simulink library "bcm"  (R2021b)
settings: Solver=VariableStepAuto  StartTime=0.0  StopTime=10.0  RelTol=1e-3
undefined symbols (not defined in the file or in its folder): ENUM_ANTITHEFT_ALARM, ENUM_ANTITHEFT_ARM, ENUM_ANTITHEFT_DISARM, ENUM_ANTITHEFT_WAIT, ENUM_GEARPOSNTOCAN_P, ENUM_PDKEYRAWLULOCK_INUNLOCK, ENUM_PDKEYRAWPS_INPS, ENUM_POWERSTA_READY, ENUM_POWERSTA_STANDBY, FALSE, KBCM_ALMBrightnessDark_enum, KBCM_AmbBlue_enum, KBCM_AmbBreathT_K, KBCM_AmbBreathTOut_K, KBCM_AmbGreen_enum, KBCM_AmbLightUser_enum, KBCM_AmbPreset_enum, KBCM_AmbRed_enum, KBCM_Antitheft_enum_ovrdflg, KBCM_Antitheft_enum_ovrdval, KBCM_APMDoorCtrlSta_flg_ovrdflg, KBCM_APMDoorCtrlSta_flg_ovrdval, KBCM_DelayTSW_flg, KBCM_DiagFLTC_mA, KBCM_DiagFMHT_s, KBCM_DiagFRTC_mA, KBCM_DiagRLTC_mA, KBCM_DiagRRTC_mA, KBCM_DrAPMRetryTimes_cnt, KBCM_DrOpenWdwOT_s, KBCM_DrOpenWdwReady_s, KBCM_ESSOffT_ms, KBCM_ESSOnT_ms, KBCM_IVIRstHoldT_ms, KBCM_IVIRstTriggerT_ms, KBCM_ONDelayT_ms, KBCM_ReDetectT_K, KBCM_RmLampKeep_min, KBCM_RmLpKeyInT_s, KBCM_RmLpKeyMissT_s, KBCM_SlpDebounceTime_s, KBCM_SPTGDetectT_sec, KBCM_SPTGLeave_flg, KBCM_SPTGLeftBound_cm, KBCM_SPTGLeftBoundOut_cm, KBCM_SPTGLowerBound_cm, KBCM_SPTGLowerBoundOut_cm, KBCM_SPTGRightBound_cm, KBCM_SPTGRightBoundOut_cm, KBCM_SPTGTOut_K, KBCM_SPTGUpperBound_cm, KBCM_SPTGUpperBoundOut_cm, KBCM_SPTGWaitDKC_sec, KBCM_USSDis_cm, KBCM_USSFilterT_K, KBCM_WaitAPMPwr_K, KBCM_WdwManualDetT_s, MIN2SEC, TRUE, XX2KXX
libraries: simulink x41, $bdroot x3, hcu_lib x2
(part 2 of 6)

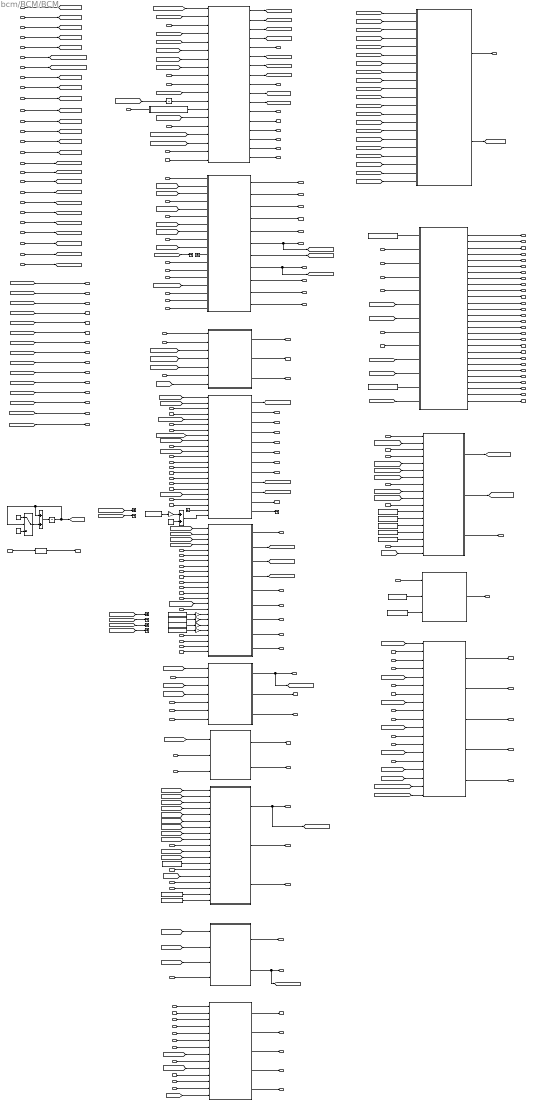
== system bcm/BCM/BCM ==
  task_time_s : Inport
  VINP_VehSpeed_kph : Inport  Port=2
  VINP_AirBagFailCmd_flg : Inport  Port=3
  VINP_ActBrkLampSta_flg : Inport  Port=4
  VINP_SRRODAWarnR_flg : Inport  Port=5
  VINP_SRRODAWarnL_flg : Inport  Port=6
  VINP_SRRBSDWarnR_flg : Inport  Port=7
  VINP_SRRBSDWarnL_flg : Inport  Port=8
  VINP_ESSActive_flg : Inport  Port=9
  VINP_LeftTurnReq_flg : Inport  Port=10
  VINP_RightTurnReq_flg : Inport  Port=11
  VINP_ForceLowBeam_enum : Inport  Port=12
  VINP_HazardWarningReq_flg : Inport  Port=13
  VINP_SetUnlockSingle_flg : Inport  Port=14
  VINP_IVIStatus_flg : Inport  Port=15
  VINP_IVINightModeSta_flg : Inport  Port=16
  VINP_HeadLampSW_enum : Inport  Port=17
  VINP_RFogLampSW_flg : Inport  Port=18
  VINP_FollowMeSW_flg : Inport  Port=19
  VINP_IVIRRDefReq_flg : Inport  Port=20
  VINP_IVIWIMAINSW_flg : Inport  Port=21
  VINP_CANMsgValidIVI2_flg : Inport  Port=22
  VINP_CDLUnlockButt_flg : Inport  Port=23  OutDataTypeStr=boolean
  VINP_CDLLockButt_flg : Inport  Port=24  OutDataTypeStr=boolean
  VINP_RoomLampMode_flg : Inport  Port=25
  VINP_MFRDNBrightReq_pct : Inport  Port=26
  VINP_METERKPHCalcu_kph : Inport  Port=27
  VINP_IVIPWModeReq_enum : Inport  Port=28
  VINP_LINKtoDrive_flg : Inport  Port=29
  VINP_AmbLightColorSet_enum : Inport  Port=30
  VINP_AmbLightUserSet_enum : Inport  Port=31
  VINP_DRAmbLightBrightnessSet_pct : Inport  Port=32
  VINP_IPAmbLightBrightnessSet_pct : Inport  Port=33
  VINP_IVIPTGUSStaSW_flg : Inport  Port=34
  VINP_LDrvControlCommand_pct : Inport  Port=35
  VINP_LPasControlCommand_pct : Inport  Port=36
  VINP_LRLDControlCommand_pct : Inport  Port=37
  VINP_LRRDControlCommand_pct : Inport  Port=38
  VINP_OpenDrOpenWdoSW_flg : Inport  Port=39
  VINP_IVILockSoundSWSta_flg : Inport  Port=40
  VINP_AVMparkingmode_enum : Inport  Port=41
  VINP_CANMsgValidIVI1_flg : Inport  Port=42
  VINP_PCommandToBCM_enum : Inport  Port=43
  VINP_DrLockSta_flg : Inport  Port=44
  VINP_CSWDimSw_flg : Inport  Port=45
  VINP_CSWPassSWSta_flg : Inport  Port=46
  VINP_RLSLampSta_flg : Inport  Port=47
  VINP_CSWTurnSWSta_enum : Inport  Port=48
  VINP_RLTurnLampC_mA : Inport  Port=49
  VINP_RRTurnLampC_mA : Inport  Port=50
  VINP_FLTurnLampC_mA : Inport  Port=51
  VINP_FRTurnLampC_mA : Inport  Port=52
  VINP_MIRRORFOLDSW_flg : Inport  Port=53
  VINP_CSWFWasSWSta_enum : Inport  Port=54
  VINP_CSWFWipSWSta_enum : Inport  Port=55
  VINP_RLSRainSnrWiperCmd_enum : Inport  Port=56
  VINP_FWiperAS_flg : Inport  Port=57
  VINP_CSWRWipIntSwSta_enum : Inport  Port=58
  VINP_RWiperAS_flg : Inport  Port=59
  VINP_CSWRWasSWSta_enum : Inport  Port=60
  VINP_PTGRDILsta_enum : Inport  Port=61
  VINP_RWiperProtection_flg : Inport  Port=62
  VINP_FWiperProtection_flg : Inport  Port=63
  VINP_PDKeyAreaPTG_enum : Inport  Port=64
  VINP_SWCmodeSta_flg : Inport  Port=65
  VINP_CANMsgValidDKC1_flg : Inport  Port=66
  VINP_CANMsgValidGWZoneDR1_flg : Inport  Port=67
  VINP_CANMsgValidGWZoneFR1_flg : Inport  Port=68
  VINP_PTGInnerSW2_enum : Inport  Port=69
  VINP_LDrvValWdwOpened_pct : Inport  Port=70
  VINP_LPasValWdwOpened_pct : Inport  Port=71
  VINP_LRLDValWdwOpened_pct : Inport  Port=72
  VINP_LRRDValWdwOpened_pct : Inport  Port=73
  VINP_PDKeyAreaLockUnlock_enum : Inport  Port=74
  VINP_PDKeyAreaPS_enum : Inport  Port=75
  VINP_ReDoorLock_enum : Inport  Port=76
  VINP_ReOutsideMirror_enum : Inport  Port=77
  VINP_HoodSW_flg : Inport  Port=78
  VINP_TailgateSW_flg : Inport  Port=79
  VINP_DrDoorSW_flg : Inport  Port=80
  VINP_PsDoorSW_flg : Inport  Port=81
  VINP_RLDoorSW_flg : Inport  Port=82
  VINP_RRDoorSW_flg : Inport  Port=83
  VINP_TrunkHanSW_flg : Inport  Port=84
  VINP_HazardSW_flg : Inport  Port=85
  VINP_CentralDoorLockSW_flg : Inport  Port=86
  VINP_BrakeSWGPIO_flg : Inport  Port=87
  VPMM_PwrSta_enum : Inport  Port=88
  VTQD_ShiftGearPosn_enum : Inport  Port=89
  VTQD_CrashDetd_flg : Inport  Port=90
  VTQD_DiagHCrash_flg : Inport  Port=91
  VTQD_ReBrakeLPReq_flg : Inport  Port=92
  VINP_FlashAntitheft_enum : Inport  Port=93
  VINP_FlashCountAlarm_enum : Inport  Port=94
  VINP_FlashMFSWTri_flg : Inport  Port=95
  VINP_FlashMirrorFlodPos : Inport  Port=96
  VINP_FlashFuelDoorPos : Inport  Port=97
  VINP_FlashLockSetting_flg : Inport  Port=98
  VINP_FlashMFRDNBrightReq_pct : Inport  Port=99
  VINP_FlashRoomLampMode_flg : Inport  Port=100
  VINP_FlashWiperFixMode_flg : Inport  Port=101
  VINP_FlashIVIPTGUSStaSW_flg : Inport  Port=102
  VINP_FlashHoodSW_flg : Inport  Port=103
  VINP_FlashTailgateSW_flg : Inport  Port=104
  VINP_FlashCTDLockSW_flg : Inport  Port=105
  VINP_FlashTailgateHDSW_flg : Inport  Port=106
  VINP_FlashAPMDoorControlSta_flg : Inport  Port=107
  VINP_funAuto_flg : Inport  Port=108
  VINP_DiagDRLOFF_flg : Inport  Port=109
  VINP_DiagFMHT_s : Inport  Port=110
  VINP_DiagFLTC_mA : Inport  Port=111
  VINP_DiagFRTC_mA : Inport  Port=112
  VINP_DiagRLTC_mA : Inport  Port=113
  VINP_DiagRRTC_mA : Inport  Port=114
  VINP_FlashfUnlockSingle_flg : Inport  Port=115
  VAPM_PASDRMR_cm : Inport  Port=116
  VAPM_PASDRML_cm : Inport  Port=117
  VINP_APSActive_flg : Inport  Port=118
  VINP_RRDefSta_flg : Inport  Port=119
  VDDM_HVRlyOpCFS_flg : Inport  Port=120
  VDDM_MCUActCFS_flg : Inport  Port=121
  APM_Door : Subsystem
  Add1 : Sum
  AmbientLight : Subsystem
  AntiTheft : Subsystem
  BCM_WAKE_MODULE : Subsystem
  CenterDoorLock : Subsystem
  Constant10 : Constant  Value=KBCM_DelayTSW_flg
  Constant11 : Constant  Value=KBCM_ReDetectT_K
  Constant12 : Constant  Value=KBCM_SPTGDetectT_sec
  Constant13 : Constant  Value=KBCM_SPTGLeave_flg
  Constant14 : Constant  Value=KBCM_RmLampKeep_min
  Constant15 : Constant  Value=KBCM_SPTGWaitDKC_sec
  Constant16 : Constant  Value=0
  Constant17 : Constant
  Constant18 : Constant  Value=KBCM_RmLpKeyInT_s
  Constant19 : Constant  Value=KBCM_RmLpKeyMissT_s
  Constant44 : Constant  Value=KBCM_DiagFMHT_s
  Constant45 : Constant  Value=10
  Constant46 : Constant  Value=KBCM_DiagFLTC_mA
  Constant47 : Constant  Value=KBCM_DiagFRTC_mA
  Constant48 : Constant  Value=KBCM_DiagRLTC_mA
  Constant49 : Constant  Value=KBCM_DiagRRTC_mA
  Constant6 : Constant  Value=KBCM_AmbPreset_enum
  Constant7 : Constant  Value=KBCM_AmbLightUser_enum
  Constant8 : Constant  Value=KBCM_IVIRstHoldT_ms
  Constant9 : Constant  Value=KBCM_IVIRstTriggerT_ms
  Data Type Conversion : DataTypeConversion  OutDataTypeStr=uint8
  Dimmer : Subsystem
  ExteriorLight : Subsystem
  FlasherSignal : Subsystem
  Gain{,2..4} (4 alike) : Gain  Gain=10
  Gain1 : Gain  Gain=5
  Ground : Ground
  Ground1 : Ground
  IVI Reset : Subsystem
  PTG : Subsystem
  PowerMirror : Subsystem
  RearDefogger : Subsystem
  RoomLamp : Subsystem
  Sum : Sum
  Switch : Switch  Criteria=u2 > Threshold
  Tailgate : Subsystem
  Terminator{,1..7} (8 alike) : Terminator
  Unit Delay : UnitDelay  SampleTime=-1  HasFrameUpgradeWarning=on
  Unit Delay1 : UnitDelay  SampleTime=-1  HasFrameUpgradeWarning=on
  Verify : Subsystem
  WasherWiper : Subsystem
  VBCM_AntitheftSta_enum : Outport
  VBCM_TailgateRemote_enum : Outport  Port=2
  VBCM_HornCtrl_flg : Outport  Port=3
  VBCM_AllDoorSW_flg : Outport  Port=4
  VBCM_BCMDoorLockSta_flg : Outport  Port=5
  VBCM_AntitheftSeatFlod_flg : Outport  Port=6
  VBCM_HoodSW_flg : Outport  Port=7
  VBCM_TailgateSW_flg : Outport  Port=8
  VBCM_DrDoorSW_flg : Outport  Port=9
  VBCM_PsDoorSW_flg : Outport  Port=10
  VBCM_RLDoorSW_flg : Outport  Port=11
  VBCM_RRDoorSW_flg : Outport  Port=12
  VBCM_LockSetting_flg : Outport  Port=13
  VBCM_FrChargingDoorCtrl_enum : Outport  Port=14
  VBCM_RrChargingDoorCtrl_enum : Outport  Port=15
  VBCM_CrashSDetd_flg : Outport  Port=16
  VBCM_CTDCtrl_enum : Outport  Port=17
  VBCM_DoorLockIND_flg : Outport  Port=18
  VBCM_CTDLockSW_flg : Outport  Port=19
  VBCM_Dimmer_pct : Outport  Port=20
  VBCM_DimmerEN_flg : Outport  Port=21
  VBCM_PosLamp_flg : Outport  Port=22
  VBCM_LBeam_flg : Outport  Port=23
  VBCM_HBeam_flg : Outport  Port=24
  VBCM_RrFogLamp_flg : Outport  Port=25
  VBCM_BrakeLamp_flg : Outport  Port=26
  VBCM_ReverseLamp_flg : Outport  Port=27
  VBCM_LDRL_flg : Outport  Port=28
  VBCM_RDRL_flg : Outport  Port=29
  VBCM_LBSD_flg : Outport  Port=30
  VBCM_RBSD_flg : Outport  Port=31
  VBCM_HazardSW_flg : Outport  Port=32
  VBCM_LTurnLP_flg : Outport  Port=33
  VBCM_RTurnLP_flg : Outport  Port=34
  VBCM_BCMBuzzerReq_flg : Outport  Port=35
  VBCM_MirrorCtrl_enum : Outport  Port=36
  VBCM_MirrorDefog_flg : Outport  Port=37
  VBCM_RrDefog_flg : Outport  Port=38
  VBCM_RoomLampH_flg : Outport  Port=39
  VBCM_RoomLampL_flg : Outport  Port=40
  VBCM_TrunkRel_flg : Outport  Port=41
  VBCM_TailgateHDSW_flg : Outport  Port=42
  VBCM_FWiperL_flg : Outport  Port=43
  VBCM_FWiperH_flg : Outport  Port=44
  VBCM_RWiper_flg : Outport  Port=45
  VBCM_WasherCtrl_enum : Outport  Port=46
  VBCM_WiperFixMode_flg : Outport  Port=47
  VBCM_SleepReq_flg : Outport  Port=48
  VBCM_User1DrAmbLightBrightness_pct : Outport  Port=49
  VBCM_User1IPAmbLightBrightness_pct : Outport  Port=50
  VBCM_User2DrAmbLightBrightness_enum : Outport  Port=51
  VBCM_User2IPAmbLightBrightness_enum : Outport  Port=52
  VBCM_User3DrAmbLightBrightness_enum : Outport  Port=53
  VBCM_User3IPAmbLightBrightness_enum : Outport  Port=54
  VBCM_User4DrAmbLightBrightness_enum : Outport  Port=55
  VBCM_User4IPAmbLightBrightness_enum : Outport  Port=56
  VBCM_User5DrAmbLightBrightness_enum : Outport  Port=57
  VBCM_User5IPAmbLightBrightness_enum : Outport  Port=58
  VBCM_User6DrAmbLightBrightness_enum : Outport  Port=59
  VBCM_User6IPAmbLightBrightness_enum : Outport  Port=60
  VBCM_User1AmbLightColor_enum : Outport  Port=61
  VBCM_User2AmbLightColor_enum : Outport  Port=62
  VBCM_User3AmbLightColor_enum : Outport  Port=63
  VBCM_User4AmbLightColor_enum : Outport  Port=64
  VBCM_User5AmbLightColor_enum : Outport  Port=65
  VBCM_User6AmbLightColor_enum : Outport  Port=66
  VBCM_AmbLightBreath1_flg : Outport  Port=67
  VBCM_AmbLightBreath2_flg : Outport  Port=68
  VBCM_AmbLightBreath3_flg : Outport  Port=69
  VBCM_AmbLightBrightness1_enum : Outport  Port=70
  VBCM_AmbLightBrightness2_enum : Outport  Port=71
  VBCM_AmbLightBrightness3_enum : Outport  Port=72
  VBCM_AmbLightColor1_enum : Outport  Port=73
  VBCM_AmbLightColor2_enum : Outport  Port=74
  VBCM_AmbLightColor3_enum : Outport  Port=75
  VBCM_LampPwr_flg : Outport  Port=76
  VBCM_SPTGDet_flg : Outport  Port=77
  VBCM_APSOpenPTG_flg : Outport  Port=78
  VBCM_FollowMe_flg : Outport  Port=79
  VBCM_IVIRST_flg : Outport  Port=80
  VBCM_CountAlarm_enum : Outport  Port=81
  VBCM_MFSWTri_flg : Outport  Port=82
  VBCM_MirrorFlodPos_flg : Outport  Port=83
  VBCM_FuelDoorPos_flg : Outport  Port=84
  VBCM_MFRDNBrightReq_pct : Outport  Port=85
  VBCM_RoomLampMode_flg : Outport  Port=86
  VBCM_IVIPTGUSStaSW_flg : Outport  Port=87
  VBCM_PTGInnerSW2_enum : Outport  Port=88
  VBCM_DiagHCrash_flg : Outport  Port=89
  VBCM_DiagFLTS_flg : Outport  Port=90
  VBCM_DiagFRTS_flg : Outport  Port=91
  VBCM_DiagRLTS_flg : Outport  Port=92
  VBCM_DiagRRTS_flg : Outport  Port=93
  VBCM_LDrvCtrlCmd_pct : Outport  Port=94
  VBCM_LPasCtrlCmd_pct : Outport  Port=95
  VBCM_LRLDCtrlCmd_pct : Outport  Port=96
  VBCM_LRRDCtrlCmd_pct : Outport  Port=97
  VBCM_APMDoorControlSta_flg : Outport  Port=98
  VBCM_LockAlarm_enum : Outport  Port=99
  VBCM_ATCtrl_enum : Outport  Port=100
  VBCM_fUnlockSingle_flg : Outport  Port=101
  VBCM_OutMode_enum : Outport  Port=102
  wires:
  VPMM_PwrSta_enum/1 -> [VPMM_PwrSta_enum]
  VINP_TailgateSW_flg/1 -> [VINP_TailgateSW_flg]
  VINP_VehSpeed_kph/1 -> [VINP_VehSpeed_kph]
  AntiTheft/4(VBCM_AntitheftSta_enum) -> [VBCM_AntitheftSta_enum]
  AntiTheft/5(VBCM_TailgateRemote_enum) -> VBCM_TailgateRemote_enum/1
  AntiTheft/6(VBCM_HornCtrl_flg) -> [VBCM_HornCtrl_flg]
  AntiTheft/7(VBCM_AllDoorSW_flg) -> [VBCM_AllDoorSW_flg]
  AntiTheft/9(VBCM_AntitehftSeatFlod_flg) -> VBCM_AntitheftSeatFlod_flg/1
  AntiTheft/8(VBCM_BCMDoorLockSta_flg) -> [VBCM_BCMDoorLockSta_flg]
  AntiTheft/1(VBCM_ATCtrl_enum) -> [VBCM_ATCtrl_enum]
  AntiTheft/2(VBCM_ATActCtrl_enum) -> [VBCM_ATActCtrl_enum]
  AntiTheft/3(VBCM_ATAlarm_flg) -> [VBCM_ATAlarm_flg]
  CenterDoorLock/1(VBCM_LockSetting_flg) -> VBCM_LockSetting_flg/1
  CenterDoorLock/4(VBCM_CrashDetd_flg) -> VBCM_CrashSDetd_flg/1
  VINP_MFRDNBrightReq_pct/1 -> Dimmer/1(VINP_MFRDNBrightReq_pct)
  VINP_IVIStatus_flg/1 -> Dimmer/2(VINP_IVIStatus_flg)
  Dimmer/1(VBCM_Dimmer_pct) -> VBCM_Dimmer_pct/1
  Dimmer/2(VBCM_DimmerEN_flg) -> VBCM_DimmerEN_flg/1
  [VBCM_PosLamp_flg] -> Dimmer/4(VBCM_PosLamp_flag)
  [VPMM_PwrSta_enum] -> PowerMirror/1(VPMM_PwrSta_enum)
  VINP_MIRRORFOLDSW_flg/1 -> PowerMirror/2(VINP_MIRRORFOLDSW_flg)
  [VINP_VehSpeed_kph] -> PowerMirror/3(VINP_VehSpeed_kph)
  [VBCM_ATActCtrl_enum] -> PowerMirror/4(VBCM_ATActCtrl_enum)
  PowerMirror/1(VBCM_MirrorCtrl_enum) -> [VBCM_MirrorCtrl_enum], VBCM_MirrorCtrl_enum/1
  [VPMM_PwrSta_enum] -> RearDefogger/1(VPMM_PwrSta_enum)
  VINP_RRDefSta_flg/1 -> RearDefogger/2(VINP_RRDefSta_flg)
  VINP_IVIRRDefReq_flg/1 -> RearDefogger/3(VINP_IVIRRDefReq_flg)
  RearDefogger/1(VBCM_MirrorDefog_flg) -> VBCM_MirrorDefog_flg/1
  RearDefogger/2(VBCM_RrDefog_flg) -> VBCM_RrDefog_flg/1
  [VPMM_PwrSta_enum] -> RoomLamp/2(VPMM_PwrSta_enum)
  [VBCM_BCMDoorLockSta_flg] -> RoomLamp/3(VBCM_BCMDoorLockSta_flg)
  [VBCM_AllDoorSW_flg] -> RoomLamp/4(VBCM_AllDoorSW_flg)
  [VBCM_AntitheftSta_enum] -> RoomLamp/5(VBCM_AntitheftSta_enum)
  [VPMM_PwrSta_enum] -> Tailgate/1(VPMM_PwrSta_enum)
  [VINP_VehSpeed_kph] -> Tailgate/2(VINP_VehSpeed_kph)
  [VBCM_BCMDoorLockSta_flg] -> Tailgate/3(VBCM_BCMDoorLockSta_flg)
  VINP_TrunkHanSW_flg/1 -> Tailgate/4(VINP_TrunkHandleSwSG08_flg)
  Tailgate/1(VBCM_TrunkRel_flg) -> VBCM_TrunkRel_flg/1
  [VBCM_fVIGHandle_flg] -> Unit Delay/1
  VINP_RoomLampMode_flg/1 -> RoomLamp/10(VINP_RoomLampMode_flg)
  AntiTheft/10(VBCM_HoodSW_flg) -> [VBCM_HoodSW_flg]
  AntiTheft/11(VBCM_TailgateSW_flg) -> [VBCM_TailgateSW_flg]
  AntiTheft/12(VBCM_DrDoorSW_flg) -> VBCM_DrDoorSW_flg/1
  AntiTheft/13(VBCM_PsDoorSW_flg) -> VBCM_PsDoorSW_flg/1
  AntiTheft/14(VBCM_RLDoorSW_flg) -> VBCM_RLDoorSW_flg/1
  AntiTheft/15(VBCM_RRDoorSW_flg) -> VBCM_RRDoorSW_flg/1
  CenterDoorLock/8(VBCM_CTDLockSW_flg) -> [VBCM_CTDLockSW_flg], VBCM_CTDLockSW_flg/1
  Tailgate/2(VBCM_TailgateHDSW_flg) -> [VBCM_TailgateHDSW_flg], VBCM_TailgateHDSW_flg/1
  VINP_CANMsgValidIVI2_flg/1 -> [VINP_CANMsgValidIVI2_flg]
  [VINP_CANMsgValidIVI2_flg] -> RoomLamp/11(VINP_CANMsgValidIVI2_flg)
  [VINP_TailgateSW_flg] -> RoomLamp/12(VINP_TailgateSW_flg)
  CenterDoorLock/10(VBCM_DiagHCrash_flg) -> VBCM_DiagHCrash_flg/1
  [VBCM_ATCtrl_enum] -> FlasherSignal/2(VBCM_ATCtrl_enum)
  [VBCM_ATAlarm_flg] -> FlasherSignal/3(VBCM_ATAlarm_flg)
  [VPMM_PwrSta_enum] -> FlasherSignal/4(VPMM_PwrSta_enum)
  VINP_HazardSW_flg/1 -> FlasherSignal/5(VINP_HazardSW_flg)
  VINP_CSWTurnSWSta_enum/1 -> FlasherSignal/6(VINP_CSWTurnSWSta_enum)
  VINP_RLTurnLampC_mA/1 -> FlasherSignal/7(VINP_RLTurnLampC_mA)
  VINP_RRTurnLampC_mA/1 -> FlasherSignal/8(VINP_RRTurnLampC_mA)
  VINP_FLTurnLampC_mA/1 -> FlasherSignal/9(VINP_FLTurnLampC_mA)
  VINP_FRTurnLampC_mA/1 -> FlasherSignal/10(VINP_FRTurnLampC_mA)
  VINP_PTGRDILsta_enum/1 -> FlasherSignal/11(VINP_PTGRDILsta_enum)
  VINP_ESSActive_flg/1 -> FlasherSignal/12(VINP_ESSActive_flg)
  VINP_LeftTurnReq_flg/1 -> FlasherSignal/13(VINP_LeftTurnReq_flg)
  VINP_RightTurnReq_flg/1 -> FlasherSignal/14(VINP_RightTurnReq_flg)
  VINP_HazardWarningReq_flg/1 -> FlasherSignal/16(HazardWarningReq)
  FlasherSignal/1(VBCM_HazardSW_flg) -> VBCM_HazardSW_flg/1
  FlasherSignal/2(VBCM_LTurnLP_flg) -> [VBCM_LTurnLP_flg]
  task_time_s/1 -> [task_time_s]
  [VBCM_HoodSW_flg] -> BCM_WAKE_MODULE/1(VBCM_HoodSW_flg)
  [VBCM_TailgateSW_flg] -> BCM_WAKE_MODULE/2(VBCM_TailgateSW_flg)
  [VBCM_CTDLockSW_flg] -> BCM_WAKE_MODULE/3(VBCM_CTDLockSW_flg)
  [VBCM_TailgateHDSW_flg] -> BCM_WAKE_MODULE/4(VBCM_TailgateHDSW_flg)
  [VBCM_AntitheftSta_enum] -> BCM_WAKE_MODULE/5(VBCM_AntitheftSta_enum)
  [VBCM_AllDoorSW_flg] -> BCM_WAKE_MODULE/6(VBCM_AllDoorSW_flg)
  [VBCM_HornCtrl_flg] -> BCM_WAKE_MODULE/7(VBCM_HornCtrl_flg)
  [VBCM_DoorLockIND_flg] -> BCM_WAKE_MODULE/8(VBCM_DoorLockIND_flg)
  [VINP_BrakeSWGPIO_flg] -> BCM_WAKE_MODULE/9(VINP_BrakeSWGPIO_flg)
  [VBCM_PosLamp_flg] -> BCM_WAKE_MODULE/10(VBCM_PosLamp_flg)
  [VBCM_LBSD_flg] -> BCM_WAKE_MODULE/11(VBCM_LBSD_flg)
  [VBCM_RBSD_flg] -> BCM_WAKE_MODULE/12(VBCM_RBSD_flg)
  [VBCM_RTurnLP_flg] -> BCM_WAKE_MODULE/14(VBCM_RTurnLP_flg)
  [VBCM_LTurnLP_flg] -> BCM_WAKE_MODULE/13(VBCM_LTurnLP_flg)
  [VBCM_MirrorCtrl_enum] -> BCM_WAKE_MODULE/15(VBCM_MirrorCtrl_enum)
  [VBCM_RoomLampH_flg] -> BCM_WAKE_MODULE/16(VBCM_RoomLampH_flg)
  [task_time_s] -> BCM_WAKE_MODULE/17(task_time_s)
  BCM_WAKE_MODULE/1(VBCM_SleepReq_flg) -> VBCM_SleepReq_flg/1
  [VPMM_PwrSta_enum] -> ExteriorLight/2(VPMM_PwrSta_enum)
  VINP_ForceLowBeam_enum/1 -> ExteriorLight/18(VINP_ForceLowBeam_enum)
  VTQD_ReBrakeLPReq_flg/1 -> ExteriorLight/20(VTQD_ReBrakeLPReq_flg)
  VINP_METERKPHCalcu_kph/1 -> ExteriorLight/21(VINP_METERKPHCalcu_kph)
  VINP_SRRBSDWarnL_flg/1 -> ExteriorLight/17(VINP_SRRBSDWarnL_flg)
  VINP_SRRBSDWarnR_flg/1 -> ExteriorLight/16(VINP_SRRBSDWarnR_flg)
  VINP_SRRODAWarnL_flg/1 -> ExteriorLight/15(VINP_SRRODAWarnL_flg)
  VINP_SRRODAWarnR_flg/1 -> ExteriorLight/14(VINP_SRRODAWarnR_flg)
  VINP_ActBrkLampSta_flg/1 -> ExteriorLight/13(VINP_ActBrkLampSta_flg)
  VINP_RLSLampSta_flg/1 -> ExteriorLight/12(VINP_RLSLampSta_flg)
  VINP_FollowMeSW_flg/1 -> ExteriorLight/10(VINP_FollowMeSW_flg)
  VINP_CSWPassSWSta_flg/1 -> ExteriorLight/7(VINP_CSWPassSWSta_flg)
  VINP_CSWDimSw_flg/1 -> ExteriorLight/6(VINP_CSWDimSw_flg)
  VINP_RFogLampSW_flg/1 -> ExteriorLight/4(VINP_RFogLampSW_flg)
  VINP_HeadLampSW_enum/1 -> ExteriorLight/3(VINP_HeadLampSW_enum)
  [VINP_CANMsgValidIVI2_flg] -> ExteriorLight/19(VINP_CANMsgValidIVI2_flg)
  [VBCM_ATCtrl_enum] -> ExteriorLight/11(VBCM_ATCtrl_enum)
  [VBCM_OutMode_enum] -> ExteriorLight/9(VBCM_OutMode_enum)
  VINP_BrakeSWGPIO_flg/1 -> [VINP_BrakeSWGPIO_flg]
  [VINP_BrakeSWGPIO_flg] -> ExteriorLight/5(VINP_BrakeSWGPIO_flg)
  ExteriorLight/2(VBCM_LBeam_flg) -> VBCM_LBeam_flg/1
  ExteriorLight/3(VBCM_HBeam_flg) -> VBCM_HBeam_flg/1
  ExteriorLight/1(VBCM_PosLamp_flg) -> [VBCM_PosLamp_flg]
  ExteriorLight/4(VBCM_RrFogLamp_flg) -> VBCM_RrFogLamp_flg/1
  ExteriorLight/5(VBCM_BrakeLamp_flg) -> VBCM_BrakeLamp_flg/1
  ExteriorLight/6(VBCM_ReverseLamp_flg) -> VBCM_ReverseLamp_flg/1
  ExteriorLight/7(VBCM_LDRL_flg) -> VBCM_LDRL_flg/1
  ExteriorLight/8(VBCM_RDRL_flg) -> VBCM_RDRL_flg/1
  ExteriorLight/10(VBCM_RBSD_flg) -> [VBCM_RBSD_flg]
  ExteriorLight/9(VBCM_LBSD_flg) -> [VBCM_LBSD_flg]
  ExteriorLight/12(VBCM_showup_flg) -> Terminator5/1
  VINP_DrDoorSW_flg/1 -> [VINP_DrDoorSW_flg]
  VINP_IVINightModeSta_flg/1 -> [VINP_IVINightModeSta_flg]
  [VINP_IVINightModeSta_flg] -> Dimmer/3(VINP_IVINightModeSta_flg)
  [VBCM_AntitheftSta_enum] -> VBCM_AntitheftSta_enum/1
  [VBCM_HornCtrl_flg] -> VBCM_HornCtrl_flg/1
  [VBCM_AllDoorSW_flg] -> VBCM_AllDoorSW_flg/1
  [VBCM_BCMDoorLockSta_flg] -> VBCM_BCMDoorLockSta_flg/1
  [VBCM_HoodSW_flg] -> VBCM_HoodSW_flg/1
  [VBCM_TailgateSW_flg] -> VBCM_TailgateSW_flg/1
  [VINP_CANMsgValidIVI2_flg] -> Dimmer/5(VINP_CANMsgValidIVI2_flg)
  VINP_ReOutsideMirror_enum/1 -> PowerMirror/5(VINP_ReOutsideMirror_enum)
  AmbientLight/1(VBCM_User1DrAmbLightBrightness_enum) -> VBCM_User1DrAmbLightBrightness_pct/1
  AmbientLight/2(VBCM_User1IPAmbLightBrightness_enum) -> VBCM_User1IPAmbLightBrightness_pct/1
  AmbientLight/3(VBCM_User2DrAmbLightBrightness_enum) -> VBCM_User2DrAmbLightBrightness_enum/1
  AmbientLight/4(VBCM_User2IPAmbLightBrightness_enum) -> VBCM_User2IPAmbLightBrightness_enum/1
  AmbientLight/5(VBCM_User3DrAmbLightBrightness_enum) -> VBCM_User3DrAmbLightBrightness_enum/1
  AmbientLight/6(VBCM_User3IPAmbLightBrightness_enum) -> VBCM_User3IPAmbLightBrightness_enum/1
  AmbientLight/7(VBCM_User4DrAmbLightBrightness_enum) -> VBCM_User4DrAmbLightBrightness_enum/1
  AmbientLight/8(VBCM_User4IPAmbLightBrightness_enum) -> VBCM_User4IPAmbLightBrightness_enum/1
  AmbientLight/9(VBCM_User5DrAmbLightBrightness_enum) -> VBCM_User5DrAmbLightBrightness_enum/1
  AmbientLight/10(VBCM_User5IPAmbLightBrightness_enum) -> VBCM_User5IPAmbLightBrightness_enum/1
  AmbientLight/11(VBCM_User6DrAmbLightBrightness_enum) -> VBCM_User6DrAmbLightBrightness_enum/1
  AmbientLight/12(VBCM_User6IPAmbLightBrightness_enum) -> VBCM_User6IPAmbLightBrightness_enum/1
  AmbientLight/13(VBCM_User1AmbLightColor_enum) -> VBCM_User1AmbLightColor_enum/1
  AmbientLight/14(VBCM_User2AmbLightColor_enum) -> VBCM_User2AmbLightColor_enum/1
  AmbientLight/15(VBCM_User3AmbLightColor_enum) -> VBCM_User3AmbLightColor_enum/1
  AmbientLight/16(VBCM_User4AmbLightColor_enum) -> VBCM_User4AmbLightColor_enum/1
  AmbientLight/17(VBCM_User5AmbLightColor_enum) -> VBCM_User5AmbLightColor_enum/1
  AmbientLight/18(VBCM_User6AmbLightColor_enum) -> VBCM_User6AmbLightColor_enum/1
  BCM_WAKE_MODULE/2(VBCM_WakeUp_flg) -> [VBCM_WakeUp_flg]
  [VPMM_PwrSta_enum] -> AmbientLight/10(VPMM_PwrSta_enum)
  [VBCM_PosLamp_flg] -> AmbientLight/11(VBCM_PosLamp_flg)
  [VINP_DrDoorSW_flg] -> AmbientLight/7(VINP_DrDoorSW_flg)
  Constant6/1 -> AmbientLight/12(KBCM_AmbPreset_enum)
  VINP_AmbLightUserSet_enum/1 -> AmbientLight/2(VINP_AmbLightUserSet_enum)
  VINP_AmbLightColorSet_enum/1 -> AmbientLight/3(VINP_AmbLightColorSet_enum)
  VINP_LINKtoDrive_flg/1 -> AmbientLight/4(VINP_LINKtoDrive_flg)
  VINP_IPAmbLightBrightnessSet_pct/1 -> AmbientLight/8(VINP_IPAmbLightBrightnessSet_enum)
  VINP_DRAmbLightBrightnessSet_pct/1 -> AmbientLight/9(VINP_DrAmbLightBrightnessSet_enum)
  Constant7/1 -> AmbientLight/1(VINP_AmbLightUser_enum)
  [VBCM_WakeUp_flg] -> AmbientLight/13(VBCM_WakeUp_flg)
  AmbientLight/19(VBCM_AmbLightBreath1_flg) -> VBCM_AmbLightBreath1_flg/1
  AmbientLight/20(VBCM_AmbLightBreath2_flg) -> VBCM_AmbLightBreath2_flg/1
  AmbientLight/21(VBCM_AmbLightBreath3_flg) -> VBCM_AmbLightBreath3_flg/1
  AmbientLight/22(VBCM_AmbLightBrightness1_enum) -> VBCM_AmbLightBrightness1_enum/1
  AmbientLight/23(VBCM_AmbLightBrightness2_enum) -> VBCM_AmbLightBrightness2_enum/1
  AmbientLight/24(VBCM_AmbLightBrightness3_enum) -> VBCM_AmbLightBrightness3_enum/1
  AmbientLight/25(VBCM_AmbLightColor1_enum) -> VBCM_AmbLightColor1_enum/1
  AmbientLight/26(VBCM_AmbLightColor2_enum) -> VBCM_AmbLightColor2_enum/1
  AmbientLight/27(VBCM_AmbLightColor3_enum) -> VBCM_AmbLightColor3_enum/1
  AmbientLight/28(VBCM_LampPwr_flg) -> VBCM_LampPwr_flg/1
  VINP_IVIPWModeReq_enum/1 -> AmbientLight/5(VINP_IVIPWModeReq_enum)
  [VINP_IVINightModeSta_flg] -> AmbientLight/6(VINP_IVINightModeSta_flg)
  VINP_FlashAntitheft_enum/1 -> Verify/1(VINP_FlashAntitheft_enum)
  [VPMM_PwrSta_enum] -> WasherWiper/8(VPMM_PwrSta_enum)
  [VINP_CANMsgValidIVI2_flg] -> WasherWiper/10(VINP_CANMsgValidIVI2_flg)
  VINP_FWiperProtection_flg/1 -> WasherWiper/12(VINP_FWiperProtection_flg)
  VINP_CSWFWasSWSta_enum/1 -> WasherWiper/1(VINP_CSWFWasSWSta_enum)
  VINP_CSWFWipSWSta_enum/1 -> WasherWiper/2(VINP_CSWFWipSWSta_enum)
  VINP_RLSRainSnrWiperCmd_enum/1 -> WasherWiper/3(VINP_RLSRainSnrWiperCmd_enum)
  VINP_FWiperAS_flg/1 -> WasherWiper/4(VINP_FWiperAS_flg)
  VINP_CSWRWipIntSwSta_enum/1 -> WasherWiper/5(VINP_CSWRWipIntSwSta_enum)
  VINP_RWiperAS_flg/1 -> WasherWiper/6(VINP_RWiperAS_flg)
  VINP_CSWRWasSWSta_enum/1 -> WasherWiper/7(VINP_CSWRWasSWSta_enum)
  VINP_IVIWIMAINSW_flg/1 -> WasherWiper/9(VINP_IVIWIMAINSW_flg)
  VINP_RWiperProtection_flg/1 -> WasherWiper/11(VINP_RWiperProtection_flg)
  WasherWiper/1(VBCM_FrWiperL_flg) -> VBCM_FWiperL_flg/1
  WasherWiper/2(VBCM_FrWiperH_flg) -> VBCM_FWiperH_flg/1
  WasherWiper/3(VBCM_RrWiper_flg) -> VBCM_RWiper_flg/1
  WasherWiper/4(VBCM_WasherCtrl_enum) -> VBCM_WasherCtrl_enum/1
  WasherWiper/5(VBCM_WiperFixMode_flg) -> VBCM_WiperFixMode_flg/1
  PTG/2(VBCM_APSOpenPTG_flg) -> [VBCM_APSOpenPTG_flg]  "VBCM_APSOpenPTG_flg"
  [VTQD_ShiftGearPosn_enum] -> PTG/7(VTQD_ShiftGearPosn_enum)
  [VPMM_PwrSta_enum] -> PTG/6(VPMM_PwrSta_eunm)
  [VINP_VehSpeed_kph] -> PTG/10(VINP_VehSpeed_kph)
  PTG/1(VBCM_SPTGDet_flg) -> [VBCM_SPTGDet_flg]  "VBCM_SPTGDet_flg"
  VAPM_PASDRMR_cm/1 -> PTG/3(VAPM_PASDRMR_cm)
  VAPM_PASDRML_cm/1 -> PTG/4(VAPM_PASDRML_cm)
  [VINP_CANMsgValidIVI2_flg] -> PTG/9(VINP_CANMsgValidIVI2_flg)
  [VINP_PCommandToBCM_enum] -> PTG/5(VINP_PCommandToBCM_enum)
  [VINP_TailgateSW_flg] -> PTG/2(VINP_TailgateSW_flg)
  VINP_PDKeyAreaPTG_enum/1 -> PTG/1(VINP_PDKeyAreaPTG_enum)
  VINP_IVIPTGUSStaSW_flg/1 -> PTG/8(VINP_IVIPTGUSStaSW_flg)
  [VBCM_SPTGDet_flg] -> FlasherSignal/15(VINP_SPTGDet_flg)
  VTQD_ShiftGearPosn_enum/1 -> [VTQD_ShiftGearPosn_enum]
  [VTQD_ShiftGearPosn_enum] -> ExteriorLight/8(VTQD_ShiftGearPosn_enum)
  VINP_PCommandToBCM_enum/1 -> [VINP_PCommandToBCM_enum]
  Constant8/1 -> IVI Reset/2(KBCM_IVIRstHoldT_ms)
  Constant9/1 -> IVI Reset/3(KBCM_IVIRstTriggerT_ms)
  VINP_SWCmodeSta_flg/1 -> IVI Reset/1(VINP_SWCmodeSta_flg)
  IVI Reset/1(VBCM_IVIRST_flg) -> VBCM_IVIRST_flg/1
  [VBCM_APSOpenPTG_flg] -> VBCM_APSOpenPTG_flg/1
  [VBCM_SPTGDet_flg] -> VBCM_SPTGDet_flg/1
  [VBCM_PosLamp_flg] -> VBCM_PosLamp_flg/1
  ExteriorLight/11(VBCM_FollowMe_flg) -> VBCM_FollowMe_flg/1
  [VBCM_LBSD_flg] -> VBCM_LBSD_flg/1
  [VBCM_RBSD_flg] -> VBCM_RBSD_flg/1
  [VBCM_LTurnLP_flg] -> VBCM_LTurnLP_flg/1
  [VBCM_RTurnLP_flg] -> VBCM_RTurnLP_flg/1
  VDDM_MCUActCFS_flg/1 -> FlasherSignal/22(VDDM_MCUActCFS_flg)
  VDDM_HVRlyOpCFS_flg/1 -> FlasherSignal/21(VDDM_HVRlyOpCFS_flg)
  Constant14/1 -> RoomLamp/13(KBCM_RmLampKeep_min)
  VINP_FlashMFSWTri_flg/1 -> PowerMirror/6(EEP_MFSWTri_flg)
  VINP_FlashMirrorFlodPos/1 -> PowerMirror/7(EEP_MirrorFlodPos)
  PowerMirror/2(MFSWTri) -> VBCM_MFSWTri_flg/1
  PowerMirror/3(MirrorFlodPos) -> VBCM_MirrorFlodPos_flg/1
  CenterDoorLock/9(VBCM_FuelDoorPos_flg) -> VBCM_FuelDoorPos_flg/1
  AntiTheft/16(VBCM_CountAlarm_enum) -> VBCM_CountAlarm_enum/1
  Constant10/1 -> PTG/12(KBCM_DelayTSW_flg)
  Constant11/1 -> PTG/13(KBCM_ReDetectT_K)
  Constant12/1 -> PTG/14(KBCM_SPTGDetectT_sec)
  Constant13/1 -> PTG/15(KBCM_SPTGLeave_flg)
  Constant15/1 -> PTG/16(KBCM_SPTGWaitDKC_sec)
  VINP_CANMsgValidDKC1_flg/1 -> PTG/11(VINP_CANMsgValidDKC1_flg)
  VINP_FlashMFRDNBrightReq_pct/1 -> Dimmer/6(EEP_MFRDNBrightReq)
  VINP_FlashRoomLampMode_flg/1 -> RoomLamp/14(EEP_RoomLampMode)
  VINP_FlashWiperFixMode_flg/1 -> WasherWiper/13(VINP_FlashWiperFixMode)
  Dimmer/3(VBCM_MFRDNBrightReq_pct) -> VBCM_MFRDNBrightReq_pct/1
  Sum/1 -> Unit Delay1/1
  Switch/1 -> Sum/2
  Constant17/1 -> Switch/3
  Constant16/1 -> Switch/1
  Unit Delay1/1 -> [BCMInitial], Switch/2, Sum/1
  [BCMInitial] -> WasherWiper/14(BCMInitial)
  [BCMInitial] -> RoomLamp/15(BCMInitial)
  [BCMInitial] -> Dimmer/7(BCMInitial)
  [BCMInitial] -> PTG/18(BCMInitial)
  VINP_FlashIVIPTGUSStaSW_flg/1 -> PTG/17(EEP_IVIPTGUSStaSW)
  PTG/3(VBCM_IVIPTGUSStaSW_flg) -> VBCM_IVIPTGUSStaSW_flg/1
  Data Type Conversion/1 -> VBCM_PTGInnerSW2_enum/1  "VBCM_PTGInnerSW2_enum"
  VINP_PTGInnerSW2_enum/1 -> Data Type Conversion/1
  VINP_FlashHoodSW_flg/1 -> [VINP_FlashHoodSW_flg]
  VINP_FlashTailgateSW_flg/1 -> [VINP_FlashTailgateSW_flg]
  VINP_FlashCTDLockSW_flg/1 -> [VINP_FlashCTDLockSW_flg]
  VINP_FlashTailgateHDSW_flg/1 -> [VINP_FlashTailgateHDSW_flg]
  [VINP_FlashHoodSW_flg] -> BCM_WAKE_MODULE/18(VINP_FlashHoodSW_flg)
  [VINP_FlashTailgateSW_flg] -> BCM_WAKE_MODULE/19(VINP_FlashTailgateSW_flg)
  [VINP_FlashCTDLockSW_flg] -> BCM_WAKE_MODULE/20(VINP_FlashCTDLockSW_flg)
  [VINP_FlashTailgateHDSW_flg] -> BCM_WAKE_MODULE/21(VINP_FlashTailgateHDSW_flg)
  [VINP_CANMsgValidGWZoneDR1_flg] -> APM_Door/18(VINP_CANMsgValidGWZoneDR1_flg)
  [VINP_CANMsgValidGWZoneFR1_flg] -> APM_Door/19(VINP_CANMsgValidGWZoneFR1_flg)
  APM_Door/4(VBCM_LRRDCtrlCmd_pct) -> VBCM_LRRDCtrlCmd_pct/1
  APM_Door/2(VBCM_LPasCtrlCmd_pct) -> VBCM_LPasCtrlCmd_pct/1
  APM_Door/3(VBCM_LRLDCtrlCmd_pct) -> VBCM_LRLDCtrlCmd_pct/1
  [VINP_RLDoorSW_flg] -> APM_Door/11(VINP_RLDoorSW_flg)
  [VINP_DrDoorSW_flg] -> APM_Door/5(VINP_DrDoorSW_flg)
  APM_Door/5(VBCM_APMDoorControlSta_flg) -> VBCM_APMDoorControlSta_flg/1
  VINP_LRRDValWdwOpened_pct/1 -> APM_Door/13(VINP_LRRDValWdwOpened_pct)
  [VINP_CANMsgValidIVI2_flg] -> APM_Door/17(VINP_CANMsgValidIVI2_flg)
  [task_time_s] -> APM_Door/1(task_time_s)
  VINP_FlashAPMDoorControlSta_flg/1 -> APM_Door/15(VINP_FlashAPMDoorControlSta_flg)
  VINP_LPasControlCommand_pct/1 -> APM_Door/6(VINP_LPasControlCommand_pct)
  VINP_OpenDrOpenWdoSW_flg/1 -> APM_Door/2(VINP_OpenDrOpenWdoSW_flg)
  VINP_LDrvValWdwOpened_pct/1 -> APM_Door/4(VINP_LDrvValWdwOpened_pct)
  VINP_LPasValWdwOpened_pct/1 -> APM_Door/7(VINP_LPasValWdwOpened_pct)
  VINP_LRLDControlCommand_pct/1 -> APM_Door/9(VINP_LRLDControlCommand_pct)
  VINP_LRRDControlCommand_pct/1 -> APM_Door/12(VINP_LRRDControlCommand_pct)
  APM_Door/1(VBCM_LDrvCtrlCmd_pct) -> VBCM_LDrvCtrlCmd_pct/1
  [VINP_RRDoorSW_flg] -> APM_Door/14(VINP_RRDoorSW_flg)
  [VINP_PsDoorSW_flg] -> APM_Door/8(VINP_PsDoorSW_flg)
  VINP_LRLDValWdwOpened_pct/1 -> APM_Door/10(VINP_LRLDValWdwOpened_pct)
  [BCMInitial] -> APM_Door/16(BCMInitial)
  VINP_LDrvControlCommand_pct/1 -> APM_Door/3(VINP_LDrvControlCommand_pct)
  VINP_PsDoorSW_flg/1 -> [VINP_PsDoorSW_flg]
  VINP_RLDoorSW_flg/1 -> [VINP_RLDoorSW_flg]
  VINP_RRDoorSW_flg/1 -> [VINP_RRDoorSW_flg]
  VINP_CANMsgValidGWZoneDR1_flg/1 -> [VINP_CANMsgValidGWZoneDR1_flg]
  VINP_CANMsgValidGWZoneFR1_flg/1 -> [VINP_CANMsgValidGWZoneFR1_flg]
  RoomLamp/1(VBCM_RoomLampH_flg) -> [VBCM_RoomLampH_flg], VBCM_RoomLampH_flg/1
  RoomLamp/2(VBCM_RoomLampL_flg) -> VBCM_RoomLampL_flg/1
  RoomLamp/3(VBCM_RoomLampMode_flg) -> VBCM_RoomLampMode_flg/1
  [task_time_s] -> RoomLamp/1(task_time_s)
  [VINP_DrDoorSW_flg] -> RoomLamp/6(VINP_DrDoorSW_flg)
  [VINP_PsDoorSW_flg] -> RoomLamp/7(VINP_PsDoorSW_flg)
  [VINP_RLDoorSW_flg] -> RoomLamp/8(VINP_RLDoorSW_flg)
  [VINP_RRDoorSW_flg] -> RoomLamp/9(VINP_RRDoorSW_flg)
  Constant18/1 -> RoomLamp/18(KBCM_RmLpKeyInT_s)  "2400"
  VINP_PDKeyAreaLockUnlock_enum/1 -> RoomLamp/16(VINP_PDKeyAreaLockUnlock_enum)
  Constant19/1 -> RoomLamp/19(KBCM_RmLpKeyMissT_s)  "600"
  VINP_PDKeyAreaPS_enum/1 -> RoomLamp/17(VINP_PDKeyAreaPS_enum)
  VINP_DiagFLTC_mA/1 -> [VINP_DiagFLTC_mA]
  VINP_DiagFRTC_mA/1 -> [VINP_DiagFRTC_mA]
  VINP_DiagRLTC_mA/1 -> [VINP_DiagRLTC_mA]
  VINP_DiagRRTC_mA/1 -> [VINP_DiagRRTC_mA]
  VINP_funAuto_flg/1 -> [VINP_funAuto_flg]
  VINP_DiagDRLOFF_flg/1 -> [VINP_DiagDRLOFF_flg]
  VINP_DiagFMHT_s/1 -> [VINP_DiagFMHT_s]
  [task_time_s] -> ExteriorLight/1(task_time_s)
  FlasherSignal/3(VBCM_RTurnLP_flg) -> [VBCM_RTurnLP_flg]
  FlasherSignal/4(VBCM_OutMode_enum) -> [VBCM_OutMode_enum]
  FlasherSignal/5(VBCM_BCMBuzzerReq_flg) -> VBCM_BCMBuzzerReq_flg/1
  FlasherSignal/6(VBCM_DiagFLTS_flg) -> VBCM_DiagFLTS_flg/1
  FlasherSignal/7(VBCM_DiagFRTS_flg) -> VBCM_DiagFRTS_flg/1
  FlasherSignal/8(VBCM_DiagRLTS_flg) -> VBCM_DiagRLTS_flg/1
  FlasherSignal/9(VBCM_DiagRRTS_flg) -> VBCM_DiagRRTS_flg/1
  VINP_APSActive_flg/1 -> FlasherSignal/23(VINP_APSActive_flg)
  VINP_AVMparkingmode_enum/1 -> FlasherSignal/24(VINP_AVMparkingmode_enum)
  [VBCM_ATCtrl_enum] -> VBCM_ATCtrl_enum/1  "VBCM_ATCtrl_enum"
  Verify/1(VBCM_FlashAntitheft_enum) -> AntiTheft/13(VBCM_FlashAntitheft_enum)  "VBCM_FlashAntitheft_enum"
  [VINP_PCommandToBCM_enum] -> AntiTheft/1(VINP_PCommandToBCM_enum)
  [VPMM_PwrSta_enum] -> AntiTheft/2(VPMM_PwrSta_enum)
  [VINP_TailgateSW_flg] -> AntiTheft/4(VINP_TailgateSW_flg)
  [VINP_DrDoorSW_flg] -> AntiTheft/5(VINP_DrDoorSW_flg)
  [VINP_VehSpeed_kph] -> AntiTheft/11(VINP_VehSpeed_kph)
  [VBCM_APSOpenPTG_flg] -> AntiTheft/14(VINP_APSOpenPTG_flg)
  [VINP_CANMsgValidGWZoneDR1_flg] -> AntiTheft/16(VINP_CANMsgValidGWZoneDR1_flg)
  [VINP_CANMsgValidGWZoneFR1_flg] -> AntiTheft/17(VINP_CANMsgValidGWZoneFR1_flg)
  [VINP_PsDoorSW_flg] -> AntiTheft/6(VINP_PsDoorSW_flg)
  [VINP_RLDoorSW_flg] -> AntiTheft/7(VINP_RLDoorSW_flg)
  [VINP_RRDoorSW_flg] -> AntiTheft/8(VINP_RRDoorSW_flg)
  Unit Delay/1 -> AntiTheft/12(VBCM_fVIGHandle_flg)
  VINP_HoodSW_flg/1 -> AntiTheft/3(VINP_HoodSW_flg)
  VINP_DrLockSta_flg/1 -> AntiTheft/9(VINP_DrLockSta_flg)
  VINP_ReDoorLock_enum/1 -> AntiTheft/10(VINP_ReDoorLock_enum)
  VINP_FlashCountAlarm_enum/1 -> AntiTheft/15(VINP_FlashCountAlarm_enum)
  AntiTheft/17(VBCM_LockAlarm_enum) -> VBCM_LockAlarm_enum/1
  VINP_IVILockSoundSWSta_flg/1 -> AntiTheft/19(VINP_IVILockSoundSWSta_flg)
  VINP_CANMsgValidIVI1_flg/1 -> AntiTheft/18(VINP_CANMsgValidIVI1_flg)
  [VINP_CANMsgValidIVI2_flg] -> CenterDoorLock/15(VINP_CANMsgValidIVI2_flg)
  [VBCM_AntitheftSta_enum] -> CenterDoorLock/2(VBCM_AntitheftSta_enum)
  [VBCM_AllDoorSW_flg] -> CenterDoorLock/3(VBCM_AllDoorSW_flg)
  [VPMM_PwrSta_enum] -> CenterDoorLock/5(VPMM_PwrSta_enum)
  [VBCM_BCMDoorLockSta_flg] -> CenterDoorLock/7(VBCM_BCMDoorLockSta_flg)
  [VBCM_ATActCtrl_enum] -> CenterDoorLock/8(VBCM_ATActCtrl_enum)
  [VINP_VehSpeed_kph] -> CenterDoorLock/10(VINP_VehSpeed_kph)
  VINP_SetUnlockSingle_flg/1 -> CenterDoorLock/1(VINP_SetUnlockSingle_flg)
  VTQD_DiagHCrash_flg/1 -> CenterDoorLock/4(VTQD_DiagHCrash_flg)
  VINP_CentralDoorLockSW_flg/1 -> CenterDoorLock/6(VINP_CentralDoorLockSW_flg)
  VINP_AirBagFailCmd_flg/1 -> CenterDoorLock/9(VINP_AirBagFailCmd_flg)
  VINP_CDLUnlockButt_flg/1 -> CenterDoorLock/12(VINP_CDLUnlockButt_flg)
  VINP_CDLLockButt_flg/1 -> CenterDoorLock/13(VINP_CDLLockButt_flg)
  VTQD_CrashDetd_flg/1 -> CenterDoorLock/14(VTQD_CrashDetd_flg)
  VINP_FlashFuelDoorPos/1 -> CenterDoorLock/16(EEP_FuelDoorPos)
  VINP_FlashLockSetting_flg/1 -> CenterDoorLock/17(EEP_LockSetting)
  CenterDoorLock/3(VBCM_RrChargingDoorCtrl_enum) -> VBCM_RrChargingDoorCtrl_enum/1
  CenterDoorLock/2(VBCM_FrChargingDoorCtrl_enum) -> VBCM_FrChargingDoorCtrl_enum/1
  CenterDoorLock/5(VBCM_CTDCtrl_enum) -> VBCM_CTDCtrl_enum/1
  CenterDoorLock/6(DoorLockIND) -> VBCM_DoorLockIND_flg/1, [VBCM_DoorLockIND_flg]
  CenterDoorLock/7(VBCM_fVIGHandle_flg) -> [VBCM_fVIGHandle_flg]
  CenterDoorLock/11(VBCM_fUnlockSingle_flg) -> VBCM_fUnlockSingle_flg/1
  VINP_FlashfUnlockSingle_flg/1 -> CenterDoorLock/18(VINP_FlashfUnlockSingle_flg)
  [task_time_s] -> FlasherSignal/1(task_time_s)
  [VINP_funAuto_flg] -> Terminator/1
  Ground/1 -> CenterDoorLock/11(VINP_funAuto_flg)
  [VINP_DiagDRLOFF_flg] -> Terminator1/1
  [VINP_DiagFMHT_s] -> Terminator2/1
  Ground1/1 -> ExteriorLight/22(VINP_DiagDRLOFF_flg)
  Gain1/1 -> Add1/1
  Constant44/1 -> Gain1/1
  Constant45/1 -> Add1/2
  Add1/1 -> ExteriorLight/23(VINP_DiagFMHT_s)
  [VINP_DiagFLTC_mA] -> Terminator3/1
  [VINP_DiagFRTC_mA] -> Terminator4/1
  [VINP_DiagRLTC_mA] -> Terminator6/1
  [VINP_DiagRRTC_mA] -> Terminator7/1
  Constant47/1 -> Gain2/1
  Constant48/1 -> Gain3/1
  Gain/1 -> FlasherSignal/17(VBCM_DiagFLTC_mA)
  Gain4/1 -> FlasherSignal/20(VBCM_DiagRRTC_mA)
  Constant49/1 -> Gain4/1
  Gain2/1 -> FlasherSignal/18(VBCM_DiagFRTC_mA)
  Constant46/1 -> Gain/1
  Gain3/1 -> FlasherSignal/19(VBCM_DiagRLTC_mA)
  [VBCM_OutMode_enum] -> VBCM_OutMode_enum/1

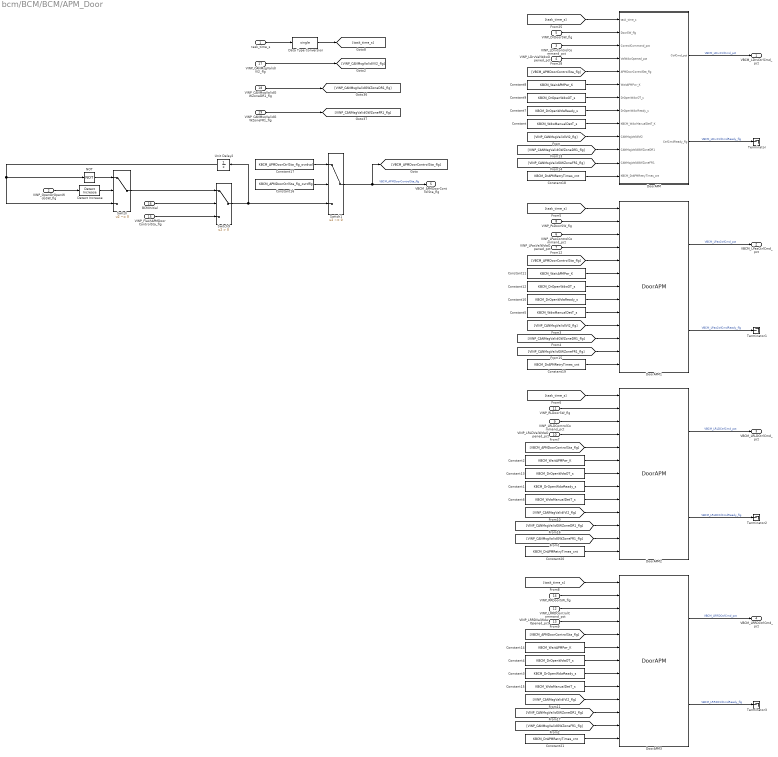
== system bcm/BCM/BCM/APM_Door ==
  task_time_s : Inport
  VINP_OpenDrOpenWdoSW_flg : Inport  Port=2
  VINP_LDrvControlCommand_pct : Inport  Port=3
  VINP_LDrvValWdwOpened_pct : Inport  Port=4
  VINP_DrDoorSW_flg : Inport  Port=5
  VINP_LPasControlCommand_pct : Inport  Port=6
  VINP_LPasValWdwOpened_pct : Inport  Port=7
  VINP_PsDoorSW_flg : Inport  Port=8
  VINP_LRLDControlCommand_pct : Inport  Port=9
  VINP_LRLDValWdwOpened_pct : Inport  Port=10
  VINP_RLDoorSW_flg : Inport  Port=11
  VINP_LRRDControlCommand_pct : Inport  Port=12
  VINP_LRRDValWdwOpened_pct : Inport  Port=13
  VINP_RRDoorSW_flg : Inport  Port=14
  VINP_FlashAPMDoorControlSta_flg : Inport  Port=15
  BCMInitial : Inport  Port=16
  VINP_CANMsgValidIVI2_flg : Inport  Port=17
  VINP_CANMsgValidGWZoneDR1_flg : Inport  Port=18
  VINP_CANMsgValidGWZoneFR1_flg : Inport  Port=19
  Constant{,5..6,15} (4 alike) : Constant  Value=KBCM_WdwManualDetT_s
  Constant{1,3,7,10} (4 alike) : Constant  Value=KBCM_DrOpenWdwReady_s
  Constant{2,8,11,14} (4 alike) : Constant  Value=KBCM_WaitAPMPwr_K
  Constant{4,9,12..13} (4 alike) : Constant  Value=KBCM_DrOpenWdwOT_s
  Constant16 : Constant  Value=KBCM_APMDoorCtrlSta_flg_ovrdflg
  Constant17 : Constant  Value=KBCM_APMDoorCtrlSta_flg_ovrdval
  Constant{18..21} (4 alike) : Constant  Value=KBCM_DrAPMRetryTimes_cnt
  Data Type Conversion : DataTypeConversion  OutDataTypeStr=single
  Detect Increase : simulink/Logic and Bit Operations/Detect Increase  vinit=0.0  OutDataTypeStr=boolean
  DoorAPM : Subsystem
  DoorAPM1 : $bdroot/BCM/BCM/APM_Door/DoorAPM  SystemSampleTime=-1  VariantActivationTime=update diagram  Latency=0  AutoFrameSizeCalculation=off
  DoorAPM2 : $bdroot/BCM/BCM/APM_Door/DoorAPM  SystemSampleTime=-1  VariantActivationTime=update diagram  Latency=0  AutoFrameSizeCalculation=off
  DoorAPM3 : $bdroot/BCM/BCM/APM_Door/DoorAPM  SystemSampleTime=-1  VariantActivationTime=update diagram  Latency=0  AutoFrameSizeCalculation=off
  NOT : Logic  Operator=NOT  AllPortsSameDT=off  OutDataTypeStr=boolean
  Switch : Switch  Criteria=u2 ~= 0
  Switch1 : Switch  Criteria=u2 ~= 0
  Switch9 : Switch  Criteria=u2 > Threshold
  Terminator{,1..3} (4 alike) : Terminator
  Unit Delay2 : UnitDelay  InitialCondition=1  SampleTime=-1  HasFrameUpgradeWarning=on
  VBCM_LDrvCtrlCmd_pct : Outport
  VBCM_LPasCtrlCmd_pct : Outport  Port=2
  VBCM_LRLDCtrlCmd_pct : Outport  Port=3
  VBCM_LRRDCtrlCmd_pct : Outport  Port=4
  VBCM_APMDoorControlSta_flg : Outport  Port=5
  wires:
  NOT/1 -> Switch/1
  VINP_OpenDrOpenWdoSW_flg/1 -> Detect Increase/1
  Detect Increase/1 -> Switch/2
  VINP_FlashAPMDoorControlSta_flg/1 -> Switch9/3
  Unit Delay2/1 -> NOT/1, Switch/3
  Switch/1 -> Switch9/1
  Switch9/1 -> Switch1/3, Unit Delay2/1
  task_time_s/1 -> Data Type Conversion/1
  [task_time_s] -> DoorAPM/1(task_time_s)
  [task_time_s] -> DoorAPM1/1
  [task_time_s] -> DoorAPM2/1
  [task_time_s] -> DoorAPM3/1
  DoorAPM/1(CtrlCmd_pct) -> VBCM_LDrvCtrlCmd_pct/1  "VBCM_LDrvCtrlCmd_pct"
  DoorAPM1/1 -> VBCM_LPasCtrlCmd_pct/1  "VBCM_LPasCtrlCmd_pct"
  DoorAPM2/1 -> VBCM_LRLDCtrlCmd_pct/1  "VBCM_LRLDCtrlCmd_pct"
  DoorAPM3/1 -> VBCM_LRRDCtrlCmd_pct/1  "VBCM_LRRDCtrlCmd_pct"
  DoorAPM/2(CtrlCmdReady_flg) -> Terminator/1  "VBCM_LDrvCtrlCmdReady_flg"
  DoorAPM1/2 -> Terminator1/1  "VBCM_LPasCtrlCmdReady_flg"
  DoorAPM2/2 -> Terminator2/1  "VBCM_LRLDCtrlCmdReady_flg"
  DoorAPM3/2 -> Terminator3/1  "VBCM_LRRDCtrlCmdReady_flg"
  Switch1/1 -> [VBCM_APMDoorControlSta_flg], VBCM_APMDoorControlSta_flg/1  "VBCM_APMDoorControlSta_flg"
  Constant16/1 -> Switch1/2
  Constant17/1 -> Switch1/1
  VINP_CANMsgValidIVI2_flg/1 -> [VINP_CANMsgValidIVI2_flg]
  VINP_CANMsgValidGWZoneDR1_flg/1 -> [VINP_CANMsgValidGWZoneDR1_flg]
  VINP_CANMsgValidGWZoneFR1_flg/1 -> [VINP_CANMsgValidGWZoneFR1_flg]
  [VINP_CANMsgValidGWZoneFR1_flg] -> DoorAPM/12(CANMsgValidGWZoneFR1)
  [VINP_CANMsgValidGWZoneDR1_flg] -> DoorAPM/11(CANMsgValidGWZoneDR1)
  [VBCM_APMDoorControlSta_flg] -> DoorAPM/5(APMDoorControlSta_flg)
  Constant8/1 -> DoorAPM/6(WaitAPMPwr_K)
  Constant9/1 -> DoorAPM/7(DrOpenWdwOT_s)
  Constant7/1 -> DoorAPM/8(DrOpenWdwReady_s)
  Constant18/1 -> DoorAPM/13(KBCM_DrAPMRetryTimes_cnt)
  Constant/1 -> DoorAPM/9(KBCM_WdwManualDetT_K)
  [VINP_CANMsgValidIVI2_flg] -> DoorAPM/10(CANMsgValidIVI2)
  VINP_DrDoorSW_flg/1 -> DoorAPM/2(DoorSW_flg)
  VINP_LDrvControlCommand_pct/1 -> DoorAPM/3(ControlCommand_pct)
  VINP_LDrvValWdwOpened_pct/1 -> DoorAPM/4(ValWdwOpened_pct)
  [VINP_CANMsgValidGWZoneDR1_flg] -> DoorAPM1/11
  [VINP_CANMsgValidGWZoneFR1_flg] -> DoorAPM1/12
  [VBCM_APMDoorControlSta_flg] -> DoorAPM1/5
  Constant11/1 -> DoorAPM1/6
  Constant12/1 -> DoorAPM1/7
  Constant10/1 -> DoorAPM1/8
  Constant5/1 -> DoorAPM1/9
  [VINP_CANMsgValidIVI2_flg] -> DoorAPM1/10
  Constant19/1 -> DoorAPM1/13
  VINP_PsDoorSW_flg/1 -> DoorAPM1/2
  VINP_LPasControlCommand_pct/1 -> DoorAPM1/3
  VINP_LPasValWdwOpened_pct/1 -> DoorAPM1/4
  [VINP_CANMsgValidGWZoneDR1_flg] -> DoorAPM2/11
  [VINP_CANMsgValidGWZoneFR1_flg] -> DoorAPM2/12
  [VBCM_APMDoorControlSta_flg] -> DoorAPM2/5
  Constant2/1 -> DoorAPM2/6
  Constant13/1 -> DoorAPM2/7
  Constant1/1 -> DoorAPM2/8
  Constant6/1 -> DoorAPM2/9
  [VINP_CANMsgValidIVI2_flg] -> DoorAPM2/10
  Constant20/1 -> DoorAPM2/13
  VINP_RLDoorSW_flg/1 -> DoorAPM2/2
  VINP_LRLDControlCommand_pct/1 -> DoorAPM2/3
  VINP_LRLDValWdwOpened_pct/1 -> DoorAPM2/4
  [VINP_CANMsgValidGWZoneDR1_flg] -> DoorAPM3/11
  [VINP_CANMsgValidGWZoneFR1_flg] -> DoorAPM3/12
  [VBCM_APMDoorControlSta_flg] -> DoorAPM3/5
  Constant14/1 -> DoorAPM3/6
  Constant4/1 -> DoorAPM3/7
  Constant3/1 -> DoorAPM3/8
  Constant15/1 -> DoorAPM3/9
  [VINP_CANMsgValidIVI2_flg] -> DoorAPM3/10
  Constant21/1 -> DoorAPM3/13
  VINP_RRDoorSW_flg/1 -> DoorAPM3/2
  VINP_LRRDControlCommand_pct/1 -> DoorAPM3/3
  VINP_LRRDValWdwOpened_pct/1 -> DoorAPM3/4
  Data Type Conversion/1 -> [task_time_s]
  BCMInitial/1 -> Switch9/2

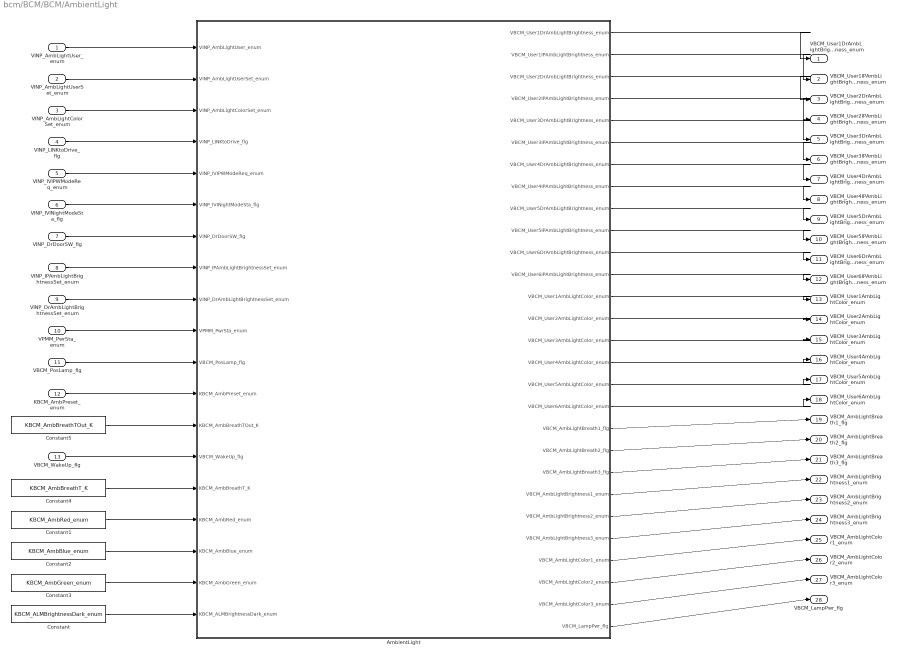
== system bcm/BCM/BCM/AmbientLight ==
  VINP_AmbLightUser_enum : Inport
  VINP_AmbLightUserSet_enum : Inport  Port=2
  VINP_AmbLightColorSet_enum : Inport  Port=3
  VINP_LINKtoDrive_flg : Inport  Port=4
  VINP_IVIPWModeReq_enum : Inport  Port=5
  VINP_IVINightModeSta_flg : Inport  Port=6
  VINP_DrDoorSW_flg : Inport  Port=7
  VINP_IPAmbLightBrightnessSet_enum : Inport  Port=8
  VINP_DrAmbLightBrightnessSet_enum : Inport  Port=9
  VPMM_PwrSta_enum : Inport  Port=10
  VBCM_PosLamp_flg : Inport  Port=11
  KBCM_AmbPreset_enum : Inport  Port=12
  VBCM_WakeUp_flg : Inport  Port=13
  AmbientLight : Stateflow chart  TreatAsAtomicUnit=on
      settings: PortSchema="{\"entries\":[{\"content\":{\"sides\":[{\"content\":{\"connectorIds\":[\"In9\",\"In2\",\"In1\",\"In6\",\"In7\",\"In11\",\"In13\",\"In15\",\"In16\",\"In14\",\"In12\",\"In17\",\"In18\",\"In19\",\"In10\",\"In5\",\"In8\",\"In4\",\"In3\"]},\"type\":\"ConnectorPlacement.EquallySpacedRectSide\",\"uuid\":\"e6ddbb92-6bab-4ee4-8600-41e59bb8ed99\"},{\"content\":{\"connectorIds\":[\"Out5\",\"Out6\",\"Out7\",\"Out8\",\"Out9\",\"Out10\",\"Out11\",\"Out12\",\"Out14\",\"Out15\",\"Out17\",\"Out18\",\"Out1\",\"Out4\",\"Out3\",\"Out2\",\"Out13\",\"Out16\",\"Out19\",\"Out20\",\"Out21\",\"Out22\",\"Out23\",\"Out24\",\"Out25\",\"Out26\",\"Out27\",\"Out28\"],\"side\":\"RIGHT\"},\"type\":\"ConnectorPlacement.EquallySpacedRectSide\",\"uuid\":\"8a02ea17-d632-4a57-b5aa-65195147745e\"},{\"content\":{\"connectorIds\":[],\"side\":\"TOP\"},\"type\":\"ConnectorPlacement.EquallySpacedRectSide\",\"uuid\":\"3394b4a4-a92c-4aad-9aa4-5f4e7dfad0c8\"}]},\"type\":\"ConnectorPlacement.EquallySpacedConnector\",\"uuid\":\"350d749b-651a-4475-8984-e64d423840e0\"}],\"packageUris\":[\"http://schema.mathworks.com/mf0/Connector/R2020b\"],\"version\":\"1.0\"}"
  Constant : Constant  Value=KBCM_ALMBrightnessDark_enum  OutDataTypeStr=uint8
  Constant1 : Constant  Value=KBCM_AmbRed_enum  OutDataTypeStr=uint8
  Constant2 : Constant  Value=KBCM_AmbBlue_enum  OutDataTypeStr=uint8
  Constant3 : Constant  Value=KBCM_AmbGreen_enum  OutDataTypeStr=uint8
  Constant4 : Constant  Value=KBCM_AmbBreathT_K  OutDataTypeStr=uint8
  Constant5 : Constant  Value=KBCM_AmbBreathTOut_K  OutDataTypeStr=uint8
  VBCM_User1DrAmbLightBrightness_enum : Outport
  VBCM_User1IPAmbLightBrightness_enum : Outport  Port=2
  VBCM_User2DrAmbLightBrightness_enum : Outport  Port=3
  VBCM_User2IPAmbLightBrightness_enum : Outport  Port=4
  VBCM_User3DrAmbLightBrightness_enum : Outport  Port=5
  VBCM_User3IPAmbLightBrightness_enum : Outport  Port=6
  VBCM_User4DrAmbLightBrightness_enum : Outport  Port=7
  VBCM_User4IPAmbLightBrightness_enum : Outport  Port=8
  VBCM_User5DrAmbLightBrightness_enum : Outport  Port=9
  VBCM_User5IPAmbLightBrightness_enum : Outport  Port=10
  VBCM_User6DrAmbLightBrightness_enum : Outport  Port=11
  VBCM_User6IPAmbLightBrightness_enum : Outport  Port=12
  VBCM_User1AmbLightColor_enum : Outport  Port=13
  VBCM_User2AmbLightColor_enum : Outport  Port=14
  VBCM_User3AmbLightColor_enum : Outport  Port=15
  VBCM_User4AmbLightColor_enum : Outport  Port=16
  VBCM_User5AmbLightColor_enum : Outport  Port=17
  VBCM_User6AmbLightColor_enum : Outport  Port=18
  VBCM_AmbLightBreath1_flg : Outport  Port=19
  VBCM_AmbLightBreath2_flg : Outport  Port=20
  VBCM_AmbLightBreath3_flg : Outport  Port=21
  VBCM_AmbLightBrightness1_enum : Outport  Port=22
  VBCM_AmbLightBrightness2_enum : Outport  Port=23
  VBCM_AmbLightBrightness3_enum : Outport  Port=24
  VBCM_AmbLightColor1_enum : Outport  Port=25
  VBCM_AmbLightColor2_enum : Outport  Port=26
  VBCM_AmbLightColor3_enum : Outport  Port=27
  VBCM_LampPwr_flg : Outport  Port=28
  wires:
  Constant4/1 -> AmbientLight/10(KBCM_AmbBreathT_K)
  Constant1/1 -> AmbientLight/5(KBCM_AmbRed_enum)
  KBCM_AmbPreset_enum/1 -> AmbientLight/17(KBCM_AmbPreset_enum)
  VBCM_PosLamp_flg/1 -> AmbientLight/12(VBCM_PosLamp_flg)
  VPMM_PwrSta_enum/1 -> AmbientLight/14(VPMM_PwrSta_enum)
  AmbientLight/16(VBCM_User6AmbLightColor_enum) -> VBCM_User6AmbLightColor_enum/1
  AmbientLight/13(VBCM_User5AmbLightColor_enum) -> VBCM_User5AmbLightColor_enum/1
  AmbientLight/2(VBCM_User4AmbLightColor_enum) -> VBCM_User4AmbLightColor_enum/1
  AmbientLight/3(VBCM_User3AmbLightColor_enum) -> VBCM_User3AmbLightColor_enum/1
  AmbientLight/4(VBCM_User2AmbLightColor_enum) -> VBCM_User2AmbLightColor_enum/1
  AmbientLight/1(VBCM_User1AmbLightColor_enum) -> VBCM_User1AmbLightColor_enum/1
  AmbientLight/18(VBCM_User6IPAmbLightBrightness_enum) -> VBCM_User6IPAmbLightBrightness_enum/1
  AmbientLight/17(VBCM_User6DrAmbLightBrightness_enum) -> VBCM_User6DrAmbLightBrightness_enum/1
  AmbientLight/15(VBCM_User5IPAmbLightBrightness_enum) -> VBCM_User5IPAmbLightBrightness_enum/1
  AmbientLight/14(VBCM_User5DrAmbLightBrightness_enum) -> VBCM_User5DrAmbLightBrightness_enum/1
  AmbientLight/12(VBCM_User4IPAmbLightBrightness_enum) -> VBCM_User4IPAmbLightBrightness_enum/1
  AmbientLight/11(VBCM_User4DrAmbLightBrightness_enum) -> VBCM_User4DrAmbLightBrightness_enum/1
  AmbientLight/10(VBCM_User3IPAmbLightBrightness_enum) -> VBCM_User3IPAmbLightBrightness_enum/1
  AmbientLight/9(VBCM_User3DrAmbLightBrightness_enum) -> VBCM_User3DrAmbLightBrightness_enum/1
  AmbientLight/8(VBCM_User2IPAmbLightBrightness_enum) -> VBCM_User2IPAmbLightBrightness_enum/1
  AmbientLight/7(VBCM_User2DrAmbLightBrightness_enum) -> VBCM_User2DrAmbLightBrightness_enum/1
  AmbientLight/6(VBCM_User1IPAmbLightBrightness_enum) -> VBCM_User1IPAmbLightBrightness_enum/1
  Constant/1 -> AmbientLight/3(KBCM_ALMBrightnessDark_enum)
  Constant3/1 -> AmbientLight/4(KBCM_AmbGreen_enum)
  Constant2/1 -> AmbientLight/8(KBCM_AmbBlue_enum)
  VINP_DrAmbLightBrightnessSet_enum/1 -> AmbientLight/16(VINP_DrAmbLightBrightnessSet_enum)
  VINP_IPAmbLightBrightnessSet_enum/1 -> AmbientLight/15(VINP_IPAmbLightBrightnessSet_enum)
  VINP_DrDoorSW_flg/1 -> AmbientLight/13(VINP_DrDoorSW_flg)
  VINP_IVINightModeSta_flg/1 -> AmbientLight/11(VINP_IVINightModeSta_flg)
  VINP_IVIPWModeReq_enum/1 -> AmbientLight/7(VINP_IVIPWModeReq_enum)
  VINP_LINKtoDrive_flg/1 -> AmbientLight/6(VINP_LINKtoDrive_flg)
  VINP_AmbLightColorSet_enum/1 -> AmbientLight/1(VINP_AmbLightColorSet_enum)
  VINP_AmbLightUserSet_enum/1 -> AmbientLight/2(VINP_AmbLightUserSet_enum)
  AmbientLight/5(VBCM_User1DrAmbLightBrightness_enum) -> VBCM_User1DrAmbLightBrightness_enum/1
  VINP_AmbLightUser_enum/1 -> AmbientLight/9(VINP_AmbLightUser_enum)
  Constant5/1 -> AmbientLight/18(KBCM_AmbBreathTOut_K)
  VBCM_WakeUp_flg/1 -> AmbientLight/19(VBCM_WakeUp_flg)
  AmbientLight/19(VBCM_AmbLightBreath1_flg) -> VBCM_AmbLightBreath1_flg/1
  AmbientLight/20(VBCM_AmbLightBreath2_flg) -> VBCM_AmbLightBreath2_flg/1
  AmbientLight/21(VBCM_AmbLightBreath3_flg) -> VBCM_AmbLightBreath3_flg/1
  AmbientLight/22(VBCM_AmbLightBrightness1_enum) -> VBCM_AmbLightBrightness1_enum/1
  AmbientLight/23(VBCM_AmbLightBrightness2_enum) -> VBCM_AmbLightBrightness2_enum/1
  AmbientLight/24(VBCM_AmbLightBrightness3_enum) -> VBCM_AmbLightBrightness3_enum/1
  AmbientLight/25(VBCM_AmbLightColor1_enum) -> VBCM_AmbLightColor1_enum/1
  AmbientLight/26(VBCM_AmbLightColor2_enum) -> VBCM_AmbLightColor2_enum/1
  AmbientLight/27(VBCM_AmbLightColor3_enum) -> VBCM_AmbLightColor3_enum/1
  AmbientLight/28(VBCM_LampPwr_flg) -> VBCM_LampPwr_flg/1
